simulink model "hw8_73S"  (R2018b)
settings: Solver=VariableStepAuto  StartTime=0.0  StopTime=2  RelTol=1e-3
values from neighbouring files (symbols this model uses):
  KI = 200    [hw8_main.m]
  KP = 108    [hw8_main.m]
settings Model: Creator=HyperDrive  LastModifiedBy=HyperDrive

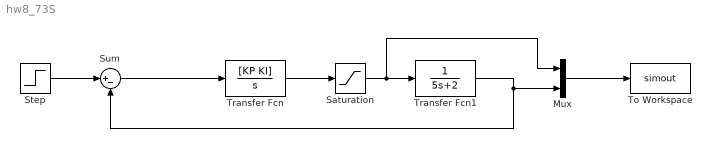
== system hw8_73S ==
  Mux : Mux  Inputs=2
  Saturation : Saturate  UpperLimit=20  LowerLimit=0
  Step : Step  Time=0  SampleTime=0
  Sum : Sum  Inputs=|+-
  To Workspace : ToWorkspace  VariableName=simout  SampleTime=-1
  Transfer Fcn : TransferFcn  Numerator=[KP KI]  Denominator=[1 0]
  Transfer Fcn1 : TransferFcn  Denominator=[5 2]
  wires:
  Saturation/1 -> Mux/1, Transfer Fcn1/1
  Step/1 -> Sum/1
  Sum/1 -> Transfer Fcn/1
  Transfer Fcn/1 -> Saturation/1
  Transfer Fcn1/1 -> Sum/2, Mux/2
  Mux/1 -> To Workspace/1
